simulink model "FullState"  (R2019b)
settings: Solver=VariableStepAuto  StartTime=0.0  StopTime=10  RelTol=1e-3
values from neighbouring files (symbols this model uses):
  K = place(Ad,Bd,P)    [PP.m]
  Nu = big_N (n+1:end,:)    [FullStateCo.m]    (also in PP.m)
  Nx = big_N(1:n,:)    [FullStateCo.m]    (also in PP.m)
  Ts = 0.05    [FullStateCo.m]    (also in LQG.m; LQRIntegalAction.m; PP.m; lin_dis.m)
undefined symbols (not defined in the file or in its folder): Ad, Bd, Cd, Dd
settings Model: Creator=elina  LastModifiedBy=elina

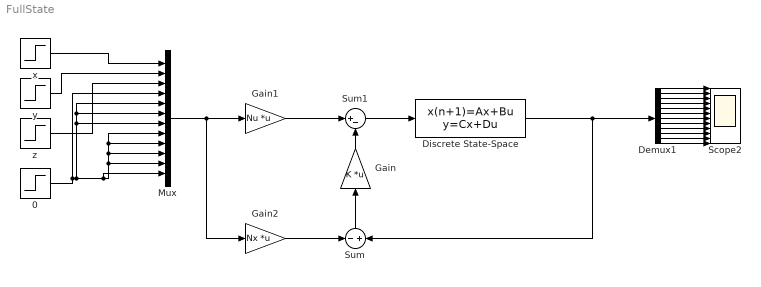
== system FullState ==
  0 : Step  Time=0  After=0  SampleTime=0
  Demux1 : Demux  Outputs=12
  Discrete State-Space : DiscreteStateSpace  A=Ad  B=Bd  C=Cd  D=Dd  SampleTime=Ts
  Gain : Gain  Gain=K  Multiplication=Matrix(K*u)
  Gain1 : Gain  Gain=Nu  Multiplication=Matrix(K*u)
  Gain2 : Gain  Gain=Nx  Multiplication=Matrix(K*u)
  Mux : Mux  Inputs=12
  Scope2 : Scope  NumInputPorts=12
  Sum : Sum  Inputs=-|+
  Sum1 : Sum  Inputs=|+-
  x : Step  SampleTime=0
  y : Step  SampleTime=0
  z : Step  SampleTime=0
  wires:
  Demux1/1 -> Scope2/1
  Demux1/2 -> Scope2/2
  Demux1/4 -> Scope2/4
  Demux1/3 -> Scope2/3
  Demux1/5 -> Scope2/5
  Demux1/6 -> Scope2/6
  Discrete State-Space/1 -> Sum/2, Demux1/1
  Demux1/7 -> Scope2/7
  Demux1/8 -> Scope2/8
  Demux1/9 -> Scope2/9
  Demux1/10 -> Scope2/10
  Demux1/11 -> Scope2/11
  Demux1/12 -> Scope2/12
  x/1 -> Mux/1
  y/1 -> Mux/2
  z/1 -> Mux/3
  0/1 -> Mux/8, Mux/9, Mux/10, Mux/11, Mux/12, Mux/5, Mux/6, Mux/7, Mux/4
  Mux/1 -> Gain2/1, Gain1/1
  Gain2/1 -> Sum/1
  Sum/1 -> Gain/1
  Gain/1 -> Sum1/2
  Gain1/1 -> Sum1/1
  Sum1/1 -> Discrete State-Space/1
